simulink model "task3_model"  (R2024a)
settings: Solver=VariableStepAuto  StartTime=0.0  StopTime=10.0  RelTol=1e-3
values from neighbouring files (symbols this model uses):
  P = motor_params()    [build_three_loop_model.m]    (also in task1_openloop.m; task2_speed_step.m; task3_lead_comp.m; task4_position_step.m)
settings Model: Creator=Prima  LastModifiedBy=Prima

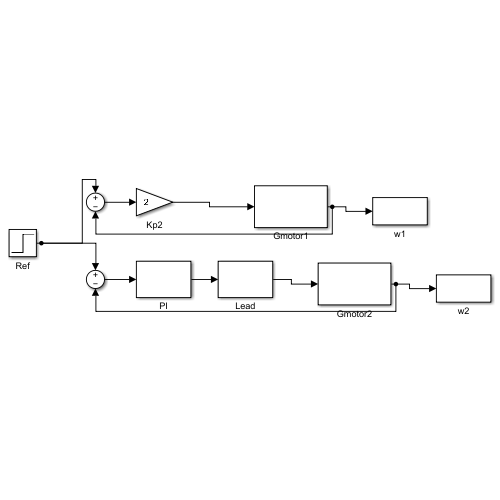
[thumbnail: Simulink's stored preview of the top-level diagram]
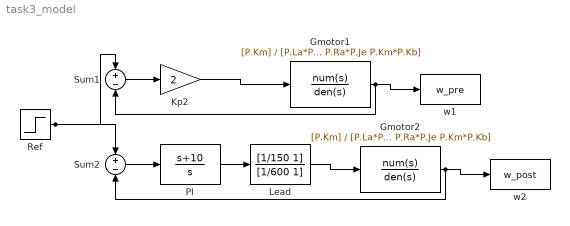
== system task3_model ==
  Gmotor1 : TransferFcn  Numerator=[P.Km]  Denominator=[P.La*P.Je P.Ra*P.Je P.Km*P.Kb]
  Gmotor2 : TransferFcn  Numerator=[P.Km]  Denominator=[P.La*P.Je P.Ra*P.Je P.Km*P.Kb]
  Kp2 : Gain  Gain=2
  Lead : TransferFcn  Numerator=[1/150 1]  Denominator=[1/600 1]
  PI : TransferFcn  Numerator=[1 10]  Denominator=[1 0]
  Ref : Step  Time=0.05  After=10  SampleTime=0
  Sum1 : Sum  Inputs=+-
  Sum2 : Sum  Inputs=+-
  w1 : ToWorkspace  VariableName=w_pre  SaveFormat=Structure With Time  SampleTime=-1
  w2 : ToWorkspace  VariableName=w_post  SaveFormat=Structure With Time  SampleTime=-1
  wires:
  Ref/1 -> Sum1/1, Sum2/1
  Sum1/1 -> Kp2/1
  Sum2/1 -> PI/1
  PI/1 -> Lead/1
  Kp2/1 -> Gmotor1/1
  Lead/1 -> Gmotor2/1
  Gmotor1/1 -> Sum1/2, w1/1
  Gmotor2/1 -> Sum2/2, w2/1
